simulink model "TST_MeUn_DD"  (R2016b)
settings: Solver=FixedStepDiscrete  StartTime=0.0  StopTime=simTime  FixedStep=sampleTime  RelTol=1e-3
values from neighbouring files (symbols this model uses):
  testCase = 1    [initTST_MeUn_DD_001.m]    (also in initTST_MeUn_DD_002.m = 2)
libraries: simulink x7, UnitTest_Lib x4
settings Model: Creator=zhengjinyan  LastModifiedBy=zhengjinyan
settings DebuggingCC: SignalRangeChecking=error

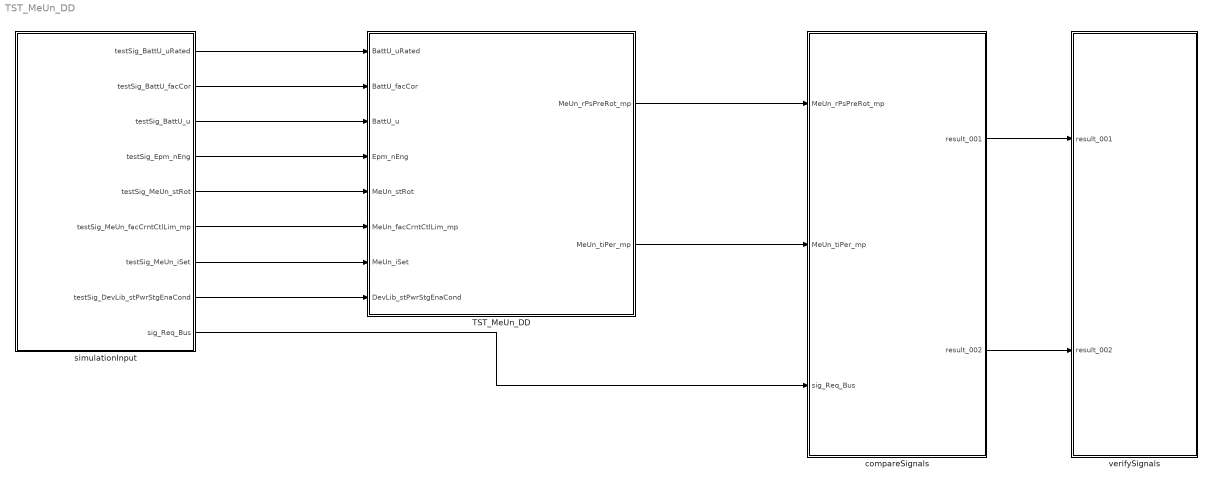
== system TST_MeUn_DD ==
  TST_MeUn_DD : Subsystem
  compareSignals : Subsystem
  simulationInput : Subsystem
  verifySignals : Subsystem
  wires:
  simulationInput/1(testSig_BattU_uRated) -> TST_MeUn_DD/1(BattU_uRated)
  simulationInput/2(testSig_BattU_facCor) -> TST_MeUn_DD/2(BattU_facCor)
  simulationInput/3(testSig_BattU_u) -> TST_MeUn_DD/3(BattU_u)
  simulationInput/4(testSig_Epm_nEng) -> TST_MeUn_DD/4(Epm_nEng)
  simulationInput/5(testSig_MeUn_stRot) -> TST_MeUn_DD/5(MeUn_stRot)
  simulationInput/6(testSig_MeUn_facCrntCtlLim_mp) -> TST_MeUn_DD/6(MeUn_facCrntCtlLim_mp)
  simulationInput/7(testSig_MeUn_iSet) -> TST_MeUn_DD/7(MeUn_iSet)
  simulationInput/8(testSig_DevLib_stPwrStgEnaCond) -> TST_MeUn_DD/8(DevLib_stPwrStgEnaCond)
  TST_MeUn_DD/1(MeUn_rPsPreRot_mp) -> compareSignals/1(MeUn_rPsPreRot_mp)
  TST_MeUn_DD/2(MeUn_tiPer_mp) -> compareSignals/2(MeUn_tiPer_mp)
  simulationInput/9(sig_Req_Bus) -> compareSignals/3(sig_Req_Bus)
  compareSignals/1(result_001) -> verifySignals/1(result_001)
  compareSignals/2(result_002) -> verifySignals/2(result_002)

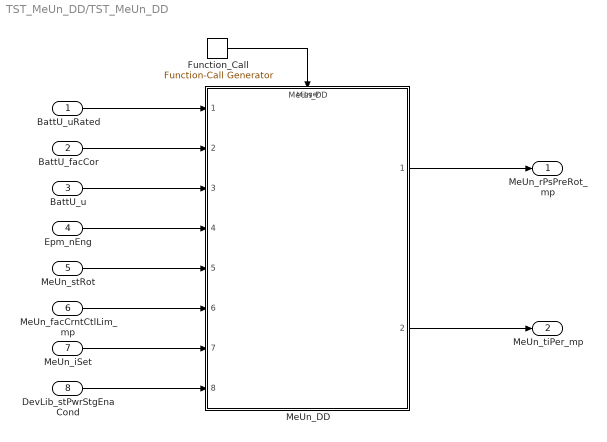
== system TST_MeUn_DD/TST_MeUn_DD ==
  BattU_uRated : Inport
  BattU_facCor : Inport  Port=2
  BattU_u : Inport  Port=3
  Epm_nEng : Inport  Port=4
  MeUn_stRot : Inport  Port=5
  MeUn_facCrntCtlLim_mp : Inport  Port=6
  MeUn_iSet : Inport  Port=7
  DevLib_stPwrStgEnaCond : Inport  Port=8
  Function_Call : simulink/Ports & Subsystems/Function-Call Generator  sample_time=sampleTime  numberOfIterations=1
  MeUn_DD : ModelReference  ModelNameDialog=MeUn_DD  SimulationMode=Normal  ModelReferenceVersion=1.26  TriggerPortName=function  TriggerPortTriggerType=function-call  TriggerPortStatesWhenEnabling=held
  MeUn_rPsPreRot_mp : Outport
  MeUn_tiPer_mp : Outport  Port=2
  wires:
  Function_Call/1 -> MeUn_DD/Trigger
  BattU_uRated/1 -> MeUn_DD/1
  BattU_facCor/1 -> MeUn_DD/2
  BattU_u/1 -> MeUn_DD/3
  Epm_nEng/1 -> MeUn_DD/4
  MeUn_stRot/1 -> MeUn_DD/5
  MeUn_facCrntCtlLim_mp/1 -> MeUn_DD/6
  MeUn_iSet/1 -> MeUn_DD/7
  DevLib_stPwrStgEnaCond/1 -> MeUn_DD/8
  MeUn_DD/1 -> MeUn_rPsPreRot_mp/1
  MeUn_DD/2 -> MeUn_tiPer_mp/1

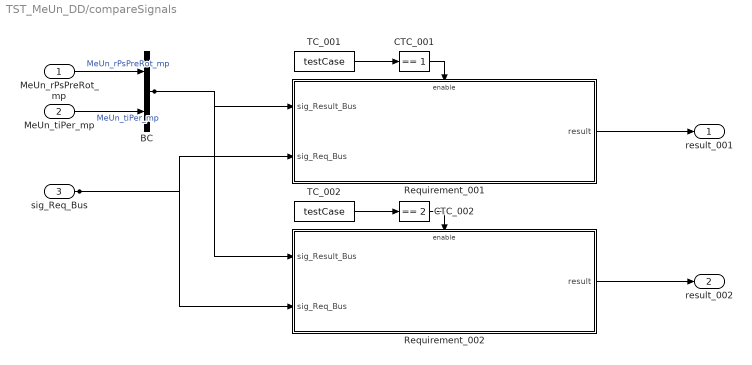
== system TST_MeUn_DD/compareSignals ==
  MeUn_rPsPreRot_mp : Inport
  MeUn_tiPer_mp : Inport  Port=2
  sig_Req_Bus : Inport  Port=3
  BC : BusCreator  Inputs=2
  CTC_001 : simulink/Logic and Bit Operations/Compare To Constant  relop===  const=1  OutDataTypeStr=boolean
  CTC_002 : simulink/Logic and Bit Operations/Compare To Constant  relop===  const=2  OutDataTypeStr=boolean
  Requirement_001 : Subsystem
  Requirement_002 : Subsystem
  TC_001 : Constant  Value=testCase
  TC_002 : Constant  Value=testCase
  result_001 : Outport
  result_002 : Outport  Port=2
  wires:
  MeUn_rPsPreRot_mp/1 -> BC/1  "MeUn_rPsPreRot_mp"
  MeUn_tiPer_mp/1 -> BC/2  "MeUn_tiPer_mp"
  TC_001/1 -> CTC_001/1
  CTC_001/1 -> Requirement_001/Enable
  sig_Req_Bus/1 -> Requirement_001/2(sig_Req_Bus), Requirement_002/2(sig_Req_Bus)
  BC/1 -> Requirement_001/1(sig_Result_Bus), Requirement_002/1(sig_Result_Bus)
  Requirement_001/1(result) -> result_001/1
  TC_002/1 -> CTC_002/1
  CTC_002/1 -> Requirement_002/Enable
  Requirement_002/1(result) -> result_002/1

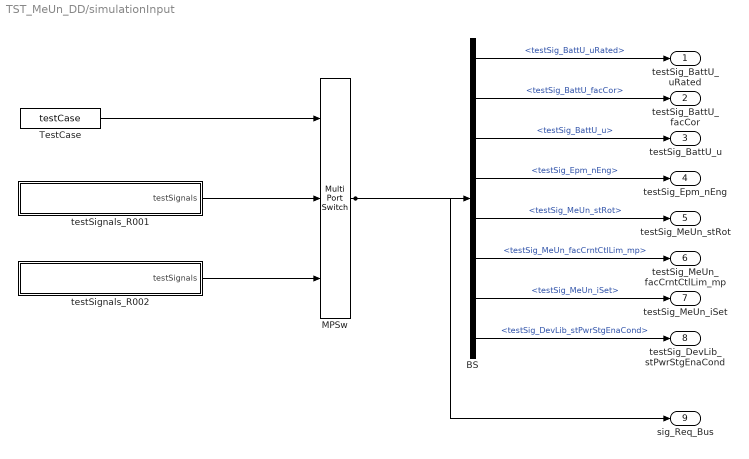
== system TST_MeUn_DD/simulationInput ==
  BS : BusSelector  OutputSignals=testSig_BattU_uRated,testSig_BattU_facCor,testSig_BattU_u,testSig_Epm_nEng,testSig_MeUn_stRot,testSig_MeUn_facCrntCtlLim_mp,testSig_MeUn_iSet,testSig_DevLib_stPwrStgEnaCond
  MPSw : MultiPortSwitch  Inputs=2  SaturateOnIntegerOverflow=on  InputSameDT=on
  TestCase : Constant  Value=testCase
  testSignals_R001 : Subsystem
  testSignals_R002 : Subsystem
  testSig_BattU_uRated : Outport
  testSig_BattU_facCor : Outport  Port=2
  testSig_BattU_u : Outport  Port=3
  testSig_Epm_nEng : Outport  Port=4
  testSig_MeUn_stRot : Outport  Port=5
  testSig_MeUn_facCrntCtlLim_mp : Outport  Port=6
  testSig_MeUn_iSet : Outport  Port=7
  testSig_DevLib_stPwrStgEnaCond : Outport  Port=8
  sig_Req_Bus : Outport  Port=9
  wires:
  BS/1 -> testSig_BattU_uRated/1  "<testSig_BattU_uRated>"
  BS/2 -> testSig_BattU_facCor/1  "<testSig_BattU_facCor>"
  BS/3 -> testSig_BattU_u/1  "<testSig_BattU_u>"
  BS/4 -> testSig_Epm_nEng/1  "<testSig_Epm_nEng>"
  BS/5 -> testSig_MeUn_stRot/1  "<testSig_MeUn_stRot>"
  BS/6 -> testSig_MeUn_facCrntCtlLim_mp/1  "<testSig_MeUn_facCrntCtlLim_mp>"
  BS/7 -> testSig_MeUn_iSet/1  "<testSig_MeUn_iSet>"
  BS/8 -> testSig_DevLib_stPwrStgEnaCond/1  "<testSig_DevLib_stPwrStgEnaCond>"
  MPSw/1 -> BS/1, sig_Req_Bus/1
  TestCase/1 -> MPSw/1
  testSignals_R001/1(testSignals) -> MPSw/2
  testSignals_R002/1(testSignals) -> MPSw/3

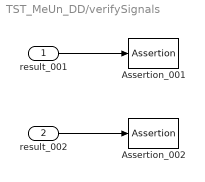
== system TST_MeUn_DD/verifySignals ==
  result_001 : Inport
  result_002 : Inport  Port=2
  Assertion_001 : Assertion  Enabled=off
  Assertion_002 : Assertion  Enabled=off
  wires:
  result_001/1 -> Assertion_001/1
  result_002/1 -> Assertion_002/1

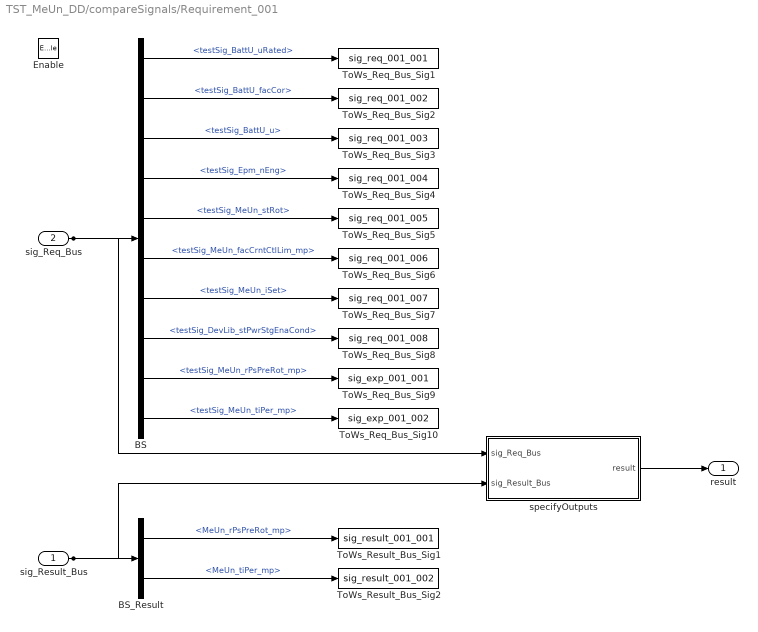
== system TST_MeUn_DD/compareSignals/Requirement_001 ==
  sig_Result_Bus : Inport
  sig_Req_Bus : Inport  Port=2
  Enable : EnablePort
  BS : BusSelector  OutputSignals=testSig_BattU_uRated,testSig_BattU_facCor,testSig_BattU_u,testSig_Epm_nEng,testSig_MeUn_stRot,testSig_MeUn_facCrntCtlLim_mp,testSig_MeUn_iSet,testSig_DevLib_stPwrStgEnaCond,testSig_MeUn_rPsPreRot_mp,testSig_MeUn_tiPer_mp
  BS_Result : BusSelector  OutputSignals=MeUn_rPsPreRot_mp,MeUn_tiPer_mp
  ToWs_Req_Bus_Sig1 : ToWorkspace  VariableName=sig_req_001_001  SaveFormat=Structure With Time
  ToWs_Req_Bus_Sig10 : ToWorkspace  VariableName=sig_exp_001_002  SaveFormat=Structure With Time
  ToWs_Req_Bus_Sig2 : ToWorkspace  VariableName=sig_req_001_002  SaveFormat=Structure With Time
  ToWs_Req_Bus_Sig3 : ToWorkspace  VariableName=sig_req_001_003  SaveFormat=Structure With Time
  ToWs_Req_Bus_Sig4 : ToWorkspace  VariableName=sig_req_001_004  SaveFormat=Structure With Time
  ToWs_Req_Bus_Sig5 : ToWorkspace  VariableName=sig_req_001_005  SaveFormat=Structure With Time
  ToWs_Req_Bus_Sig6 : ToWorkspace  VariableName=sig_req_001_006  SaveFormat=Structure With Time
  ToWs_Req_Bus_Sig7 : ToWorkspace  VariableName=sig_req_001_007  SaveFormat=Structure With Time
  ToWs_Req_Bus_Sig8 : ToWorkspace  VariableName=sig_req_001_008  SaveFormat=Structure With Time
  ToWs_Req_Bus_Sig9 : ToWorkspace  VariableName=sig_exp_001_001  SaveFormat=Structure With Time
  ToWs_Result_Bus_Sig1 : ToWorkspace  VariableName=sig_result_001_001  SaveFormat=Structure With Time
  ToWs_Result_Bus_Sig2 : ToWorkspace  VariableName=sig_result_001_002  SaveFormat=Structure With Time
  specifyOutputs : Subsystem
  result : Outport
  wires:
  sig_Req_Bus/1 -> BS/1, specifyOutputs/1(sig_Req_Bus)
  BS/1 -> ToWs_Req_Bus_Sig1/1  "<testSig_BattU_uRated>"
  BS/2 -> ToWs_Req_Bus_Sig2/1  "<testSig_BattU_facCor>"
  BS/3 -> ToWs_Req_Bus_Sig3/1  "<testSig_BattU_u>"
  BS/4 -> ToWs_Req_Bus_Sig4/1  "<testSig_Epm_nEng>"
  BS/5 -> ToWs_Req_Bus_Sig5/1  "<testSig_MeUn_stRot>"
  BS/6 -> ToWs_Req_Bus_Sig6/1  "<testSig_MeUn_facCrntCtlLim_mp>"
  BS/7 -> ToWs_Req_Bus_Sig7/1  "<testSig_MeUn_iSet>"
  BS/8 -> ToWs_Req_Bus_Sig8/1  "<testSig_DevLib_stPwrStgEnaCond>"
  BS/9 -> ToWs_Req_Bus_Sig9/1  "<testSig_MeUn_rPsPreRot_mp>"
  BS/10 -> ToWs_Req_Bus_Sig10/1  "<testSig_MeUn_tiPer_mp>"
  sig_Result_Bus/1 -> BS_Result/1, specifyOutputs/2(sig_Result_Bus)
  BS_Result/1 -> ToWs_Result_Bus_Sig1/1  "<MeUn_rPsPreRot_mp>"
  BS_Result/2 -> ToWs_Result_Bus_Sig2/1  "<MeUn_tiPer_mp>"
  specifyOutputs/1(result) -> result/1

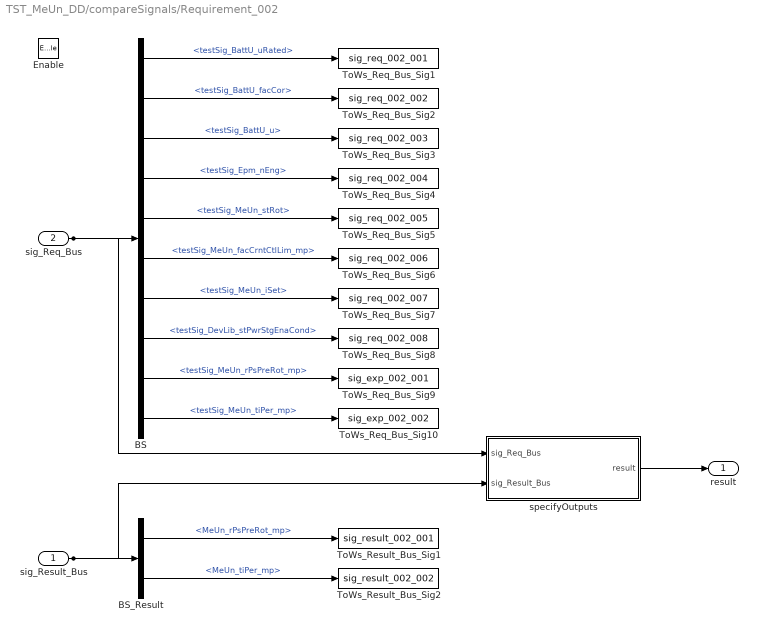
== system TST_MeUn_DD/compareSignals/Requirement_002 ==
  sig_Result_Bus : Inport
  sig_Req_Bus : Inport  Port=2
  Enable : EnablePort
  BS : BusSelector  OutputSignals=testSig_BattU_uRated,testSig_BattU_facCor,testSig_BattU_u,testSig_Epm_nEng,testSig_MeUn_stRot,testSig_MeUn_facCrntCtlLim_mp,testSig_MeUn_iSet,testSig_DevLib_stPwrStgEnaCond,testSig_MeUn_rPsPreRot_mp,testSig_MeUn_tiPer_mp
  BS_Result : BusSelector  OutputSignals=MeUn_rPsPreRot_mp,MeUn_tiPer_mp
  ToWs_Req_Bus_Sig1 : ToWorkspace  VariableName=sig_req_002_001  SaveFormat=Structure With Time
  ToWs_Req_Bus_Sig10 : ToWorkspace  VariableName=sig_exp_002_002  SaveFormat=Structure With Time
  ToWs_Req_Bus_Sig2 : ToWorkspace  VariableName=sig_req_002_002  SaveFormat=Structure With Time
  ToWs_Req_Bus_Sig3 : ToWorkspace  VariableName=sig_req_002_003  SaveFormat=Structure With Time
  ToWs_Req_Bus_Sig4 : ToWorkspace  VariableName=sig_req_002_004  SaveFormat=Structure With Time
  ToWs_Req_Bus_Sig5 : ToWorkspace  VariableName=sig_req_002_005  SaveFormat=Structure With Time
  ToWs_Req_Bus_Sig6 : ToWorkspace  VariableName=sig_req_002_006  SaveFormat=Structure With Time
  ToWs_Req_Bus_Sig7 : ToWorkspace  VariableName=sig_req_002_007  SaveFormat=Structure With Time
  ToWs_Req_Bus_Sig8 : ToWorkspace  VariableName=sig_req_002_008  SaveFormat=Structure With Time
  ToWs_Req_Bus_Sig9 : ToWorkspace  VariableName=sig_exp_002_001  SaveFormat=Structure With Time
  ToWs_Result_Bus_Sig1 : ToWorkspace  VariableName=sig_result_002_001  SaveFormat=Structure With Time
  ToWs_Result_Bus_Sig2 : ToWorkspace  VariableName=sig_result_002_002  SaveFormat=Structure With Time
  specifyOutputs : Subsystem
  result : Outport
  wires:
  sig_Req_Bus/1 -> BS/1, specifyOutputs/1(sig_Req_Bus)
  BS/1 -> ToWs_Req_Bus_Sig1/1  "<testSig_BattU_uRated>"
  BS/2 -> ToWs_Req_Bus_Sig2/1  "<testSig_BattU_facCor>"
  BS/3 -> ToWs_Req_Bus_Sig3/1  "<testSig_BattU_u>"
  BS/4 -> ToWs_Req_Bus_Sig4/1  "<testSig_Epm_nEng>"
  BS/5 -> ToWs_Req_Bus_Sig5/1  "<testSig_MeUn_stRot>"
  BS/6 -> ToWs_Req_Bus_Sig6/1  "<testSig_MeUn_facCrntCtlLim_mp>"
  BS/7 -> ToWs_Req_Bus_Sig7/1  "<testSig_MeUn_iSet>"
  BS/8 -> ToWs_Req_Bus_Sig8/1  "<testSig_DevLib_stPwrStgEnaCond>"
  BS/9 -> ToWs_Req_Bus_Sig9/1  "<testSig_MeUn_rPsPreRot_mp>"
  BS/10 -> ToWs_Req_Bus_Sig10/1  "<testSig_MeUn_tiPer_mp>"
  sig_Result_Bus/1 -> BS_Result/1, specifyOutputs/2(sig_Result_Bus)
  BS_Result/1 -> ToWs_Result_Bus_Sig1/1  "<MeUn_rPsPreRot_mp>"
  BS_Result/2 -> ToWs_Result_Bus_Sig2/1  "<MeUn_tiPer_mp>"
  specifyOutputs/1(result) -> result/1

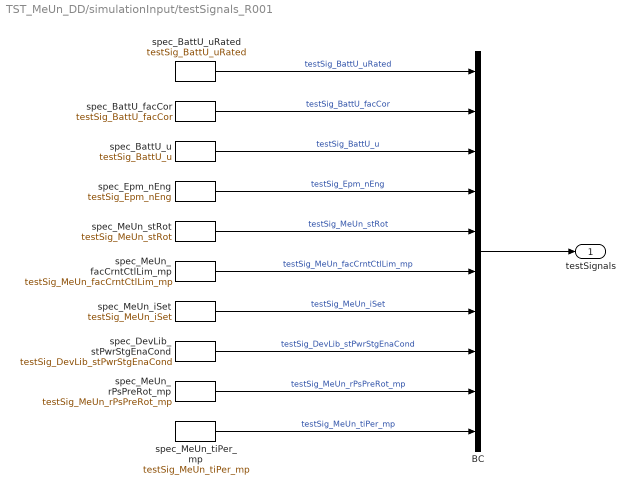
== system TST_MeUn_DD/simulationInput/testSignals_R001 ==
  BC : BusCreator  Inputs=10
  spec_BattU_facCor : FromWorkspace  VariableName=testSig_BattU_facCor  Interpolate=off  OutputAfterFinalValue=Holding final value
  spec_BattU_u : FromWorkspace  VariableName=testSig_BattU_u  Interpolate=off  OutputAfterFinalValue=Holding final value
  spec_BattU_uRated : FromWorkspace  VariableName=testSig_BattU_uRated  Interpolate=off  OutputAfterFinalValue=Holding final value
  spec_DevLib_stPwrStgEnaCond : FromWorkspace  VariableName=testSig_DevLib_stPwrStgEnaCond  Interpolate=off  OutputAfterFinalValue=Holding final value
  spec_Epm_nEng : FromWorkspace  VariableName=testSig_Epm_nEng  Interpolate=off  OutputAfterFinalValue=Holding final value
  spec_MeUn_facCrntCtlLim_mp : FromWorkspace  VariableName=testSig_MeUn_facCrntCtlLim_mp  Interpolate=off  OutputAfterFinalValue=Holding final value
  spec_MeUn_iSet : FromWorkspace  VariableName=testSig_MeUn_iSet  Interpolate=off  OutputAfterFinalValue=Holding final value
  spec_MeUn_rPsPreRot_mp : FromWorkspace  VariableName=testSig_MeUn_rPsPreRot_mp  Interpolate=off  OutputAfterFinalValue=Holding final value
  spec_MeUn_stRot : FromWorkspace  VariableName=testSig_MeUn_stRot  Interpolate=off  OutputAfterFinalValue=Holding final value
  spec_MeUn_tiPer_mp : FromWorkspace  VariableName=testSig_MeUn_tiPer_mp  Interpolate=off  OutputAfterFinalValue=Holding final value
  testSignals : Outport
  wires:
  BC/1 -> testSignals/1
  spec_BattU_uRated/1 -> BC/1  "testSig_BattU_uRated"
  spec_BattU_facCor/1 -> BC/2  "testSig_BattU_facCor"
  spec_BattU_u/1 -> BC/3  "testSig_BattU_u"
  spec_Epm_nEng/1 -> BC/4  "testSig_Epm_nEng"
  spec_MeUn_stRot/1 -> BC/5  "testSig_MeUn_stRot"
  spec_MeUn_facCrntCtlLim_mp/1 -> BC/6  "testSig_MeUn_facCrntCtlLim_mp"
  spec_MeUn_iSet/1 -> BC/7  "testSig_MeUn_iSet"
  spec_DevLib_stPwrStgEnaCond/1 -> BC/8  "testSig_DevLib_stPwrStgEnaCond"
  spec_MeUn_rPsPreRot_mp/1 -> BC/9  "testSig_MeUn_rPsPreRot_mp"
  spec_MeUn_tiPer_mp/1 -> BC/10  "testSig_MeUn_tiPer_mp"

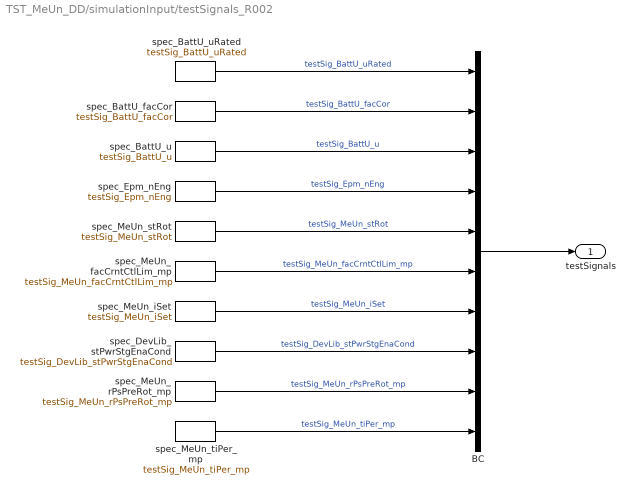
== system TST_MeUn_DD/simulationInput/testSignals_R002 ==
  BC : BusCreator  Inputs=10
  spec_BattU_facCor : FromWorkspace  VariableName=testSig_BattU_facCor  Interpolate=off  OutputAfterFinalValue=Holding final value
  spec_BattU_u : FromWorkspace  VariableName=testSig_BattU_u  Interpolate=off  OutputAfterFinalValue=Holding final value
  spec_BattU_uRated : FromWorkspace  VariableName=testSig_BattU_uRated  Interpolate=off  OutputAfterFinalValue=Holding final value
  spec_DevLib_stPwrStgEnaCond : FromWorkspace  VariableName=testSig_DevLib_stPwrStgEnaCond  Interpolate=off  OutputAfterFinalValue=Holding final value
  spec_Epm_nEng : FromWorkspace  VariableName=testSig_Epm_nEng  Interpolate=off  OutputAfterFinalValue=Holding final value
  spec_MeUn_facCrntCtlLim_mp : FromWorkspace  VariableName=testSig_MeUn_facCrntCtlLim_mp  Interpolate=off  OutputAfterFinalValue=Holding final value
  spec_MeUn_iSet : FromWorkspace  VariableName=testSig_MeUn_iSet  Interpolate=off  OutputAfterFinalValue=Holding final value
  spec_MeUn_rPsPreRot_mp : FromWorkspace  VariableName=testSig_MeUn_rPsPreRot_mp  Interpolate=off  OutputAfterFinalValue=Holding final value
  spec_MeUn_stRot : FromWorkspace  VariableName=testSig_MeUn_stRot  Interpolate=off  OutputAfterFinalValue=Holding final value
  spec_MeUn_tiPer_mp : FromWorkspace  VariableName=testSig_MeUn_tiPer_mp  Interpolate=off  OutputAfterFinalValue=Holding final value
  testSignals : Outport
  wires:
  BC/1 -> testSignals/1
  spec_BattU_uRated/1 -> BC/1  "testSig_BattU_uRated"
  spec_BattU_facCor/1 -> BC/2  "testSig_BattU_facCor"
  spec_BattU_u/1 -> BC/3  "testSig_BattU_u"
  spec_Epm_nEng/1 -> BC/4  "testSig_Epm_nEng"
  spec_MeUn_stRot/1 -> BC/5  "testSig_MeUn_stRot"
  spec_MeUn_facCrntCtlLim_mp/1 -> BC/6  "testSig_MeUn_facCrntCtlLim_mp"
  spec_MeUn_iSet/1 -> BC/7  "testSig_MeUn_iSet"
  spec_DevLib_stPwrStgEnaCond/1 -> BC/8  "testSig_DevLib_stPwrStgEnaCond"
  spec_MeUn_rPsPreRot_mp/1 -> BC/9  "testSig_MeUn_rPsPreRot_mp"
  spec_MeUn_tiPer_mp/1 -> BC/10  "testSig_MeUn_tiPer_mp"

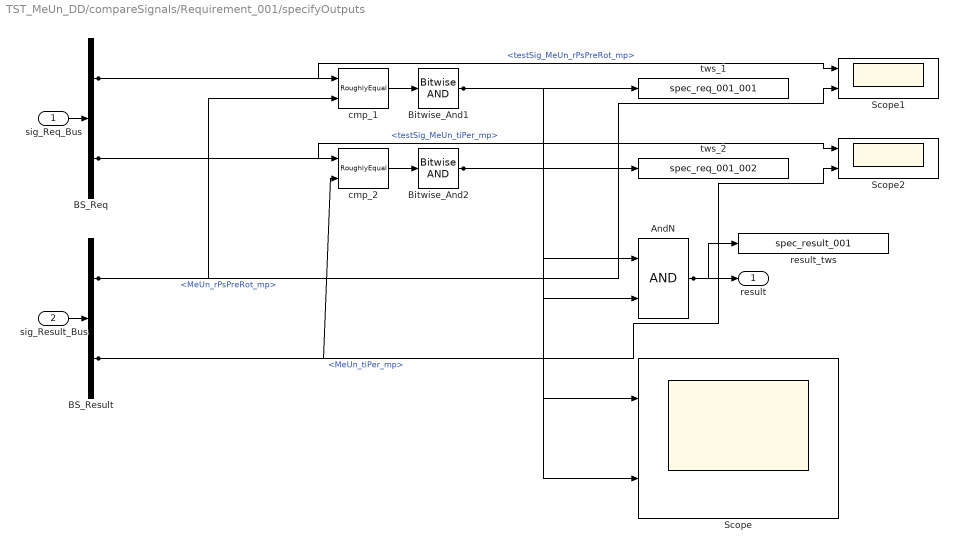
== system TST_MeUn_DD/compareSignals/Requirement_001/specifyOutputs ==
  sig_Req_Bus : Inport
  sig_Result_Bus : Inport  Port=2
  AndN : Logic
  BS_Req : BusSelector  OutputSignals=testSig_MeUn_rPsPreRot_mp,testSig_MeUn_tiPer_mp
  BS_Result : BusSelector  OutputSignals=MeUn_rPsPreRot_mp,MeUn_tiPer_mp
  Bitwise_And1 : simulink/Logic and Bit Operations/Bitwise Operator  logicop=AND  UseBitMask=off  BitMask=bin2dec('11011001')  BitMaskRealWorld=Stored Integer
  Bitwise_And2 : simulink/Logic and Bit Operations/Bitwise Operator  logicop=AND  UseBitMask=off  BitMask=bin2dec('11011001')  BitMaskRealWorld=Stored Integer
  Scope : Scope  NumInputPorts=2
  Scope1 : Scope  NumInputPorts=2
  Scope2 : Scope  NumInputPorts=2
  cmp_1 : UnitTest_Lib/RoughlyEqual  slope=0.1
  cmp_2 : UnitTest_Lib/RoughlyEqual  slope=0.1
  result_tws : ToWorkspace  VariableName=spec_result_001
  tws_1 : ToWorkspace  VariableName=spec_req_001_001
  tws_2 : ToWorkspace  VariableName=spec_req_001_002
  result : Outport
  wires:
  sig_Req_Bus/1 -> BS_Req/1
  sig_Result_Bus/1 -> BS_Result/1
  AndN/1 -> result/1, result_tws/1
  BS_Req/1 -> cmp_1/1, Scope1/1  "<testSig_MeUn_rPsPreRot_mp>"
  BS_Result/1 -> cmp_1/2, Scope1/2  "<MeUn_rPsPreRot_mp>"
  cmp_1/1 -> Bitwise_And1/1
  Bitwise_And1/1 -> tws_1/1, AndN/1, Scope/1
  BS_Req/2 -> cmp_2/1, Scope2/1  "<testSig_MeUn_tiPer_mp>"
  BS_Result/2 -> cmp_2/2, Scope2/2  "<MeUn_tiPer_mp>"
  cmp_2/1 -> Bitwise_And2/1
  Bitwise_And2/1 -> tws_2/1, AndN/2, Scope/2

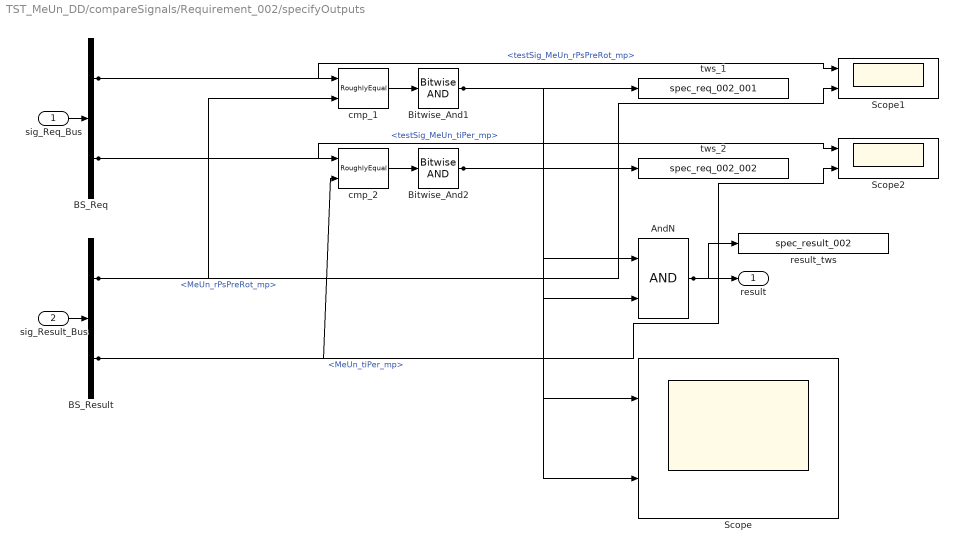
== system TST_MeUn_DD/compareSignals/Requirement_002/specifyOutputs ==
  sig_Req_Bus : Inport
  sig_Result_Bus : Inport  Port=2
  AndN : Logic
  BS_Req : BusSelector  OutputSignals=testSig_MeUn_rPsPreRot_mp,testSig_MeUn_tiPer_mp
  BS_Result : BusSelector  OutputSignals=MeUn_rPsPreRot_mp,MeUn_tiPer_mp
  Bitwise_And1 : simulink/Logic and Bit Operations/Bitwise Operator  logicop=AND  UseBitMask=off  BitMask=bin2dec('11011001')  BitMaskRealWorld=Stored Integer
  Bitwise_And2 : simulink/Logic and Bit Operations/Bitwise Operator  logicop=AND  UseBitMask=off  BitMask=bin2dec('11011001')  BitMaskRealWorld=Stored Integer
  Scope : Scope  NumInputPorts=2
  Scope1 : Scope  NumInputPorts=2
  Scope2 : Scope  NumInputPorts=2
  cmp_1 : UnitTest_Lib/RoughlyEqual  slope=0.1
  cmp_2 : UnitTest_Lib/RoughlyEqual  slope=0.1
  result_tws : ToWorkspace  VariableName=spec_result_002
  tws_1 : ToWorkspace  VariableName=spec_req_002_001
  tws_2 : ToWorkspace  VariableName=spec_req_002_002
  result : Outport
  wires:
  sig_Req_Bus/1 -> BS_Req/1
  sig_Result_Bus/1 -> BS_Result/1
  AndN/1 -> result/1, result_tws/1
  BS_Req/1 -> cmp_1/1, Scope1/1  "<testSig_MeUn_rPsPreRot_mp>"
  BS_Result/1 -> cmp_1/2, Scope1/2  "<MeUn_rPsPreRot_mp>"
  cmp_1/1 -> Bitwise_And1/1
  Bitwise_And1/1 -> tws_1/1, AndN/1, Scope/1
  BS_Req/2 -> cmp_2/1, Scope2/1  "<testSig_MeUn_tiPer_mp>"
  BS_Result/2 -> cmp_2/2, Scope2/2  "<MeUn_tiPer_mp>"
  cmp_2/1 -> Bitwise_And2/1
  Bitwise_And2/1 -> tws_2/1, AndN/2, Scope/2
